simulink model "Optimization_function"  (R2024b)
settings: Solver=VariableStepAuto  StartTime=0.0  StopTime=10.0  RelTol=1e-3
undefined symbols (not defined in the file or in its folder): alpha0, FM0, LM0
settings Model: Creator=jakub  LastModifiedBy=jakub

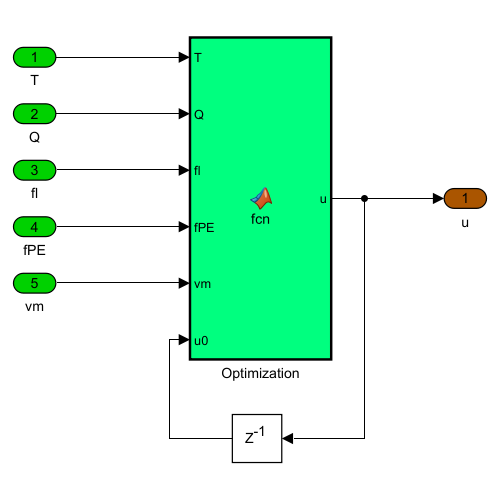
[thumbnail: Simulink's stored preview of the top-level diagram]
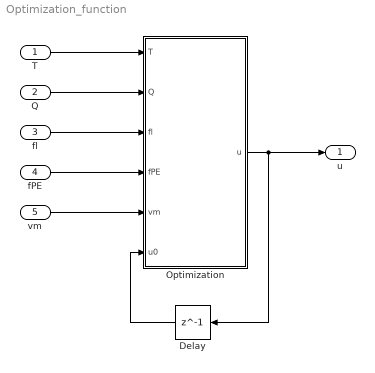
== system Optimization_function ==
  T : Inport  OutDataTypeStr=double  Unit=N*m  PortDimensions=[2 1]  SampleTime=0
  Q : Inport  Port=2  OutDataTypeStr=double  PortDimensions=[2 8]  SampleTime=0
  fl : Inport  Port=3  OutDataTypeStr=double  PortDimensions=[8 1]  SampleTime=0
  fPE : Inport  Port=4  OutDataTypeStr=double  PortDimensions=[8 1]  SampleTime=0
  vm : Inport  Port=5  OutDataTypeStr=double  Unit=m/s  PortDimensions=[8 1]  SampleTime=0
  Delay : Delay  DelayLength=1  InitialCondition=0*ones(8,1)
  Optimization : MATLAB Function  TreatAsAtomicUnit=on
  u : Outport  OutDataTypeStr=double  PortDimensions=[8 1]  SampleTime=0
  wires:
  T/1 -> Optimization/1(T)
  Delay/1 -> Optimization/6(u0)
  Optimization/1(u) -> Delay/1, u/1
  Q/1 -> Optimization/2(Q)
  fl/1 -> Optimization/3(fl)
  fPE/1 -> Optimization/4(fPE)
  vm/1 -> Optimization/5(vm)

== matlab function Optimization_function/Optimization ==
  data: u output double size=[8 1]; T input double size=[2 1]; Q input double size=[2 8]; fl input double size=[8 1]; fPE input double size=[8 1]; vm input double size=[8 1]; LM0 parameter double size=[8 1]; u0 input double size=[8 1]; alpha0 parameter; FM0 parameter
function u  = fcn(T, Q, fl, fPE, vm, LM0,u0, alpha0, FM0)
u = u0;

% coder.extrinsic('Optimization_ThelenMuscle');
% u = Optimization_ThelenMuscle(Q, T, fl, fPE, vm, LM0, u0, alpha0, FM0);

u = Optimization_ThelenMuscle_codegen(Q, T, fl, fPE, vm, LM0, u0, alpha0, FM0);



end
